simulink model "twiddle"  (R2018a)
settings: Solver=VariableStepAuto  StartTime=0.0  StopTime=10.0  RelTol=1e-3
undefined symbols (not defined in the file or in its folder): i
settings Model: Creator=berke  LastModifiedBy=berke

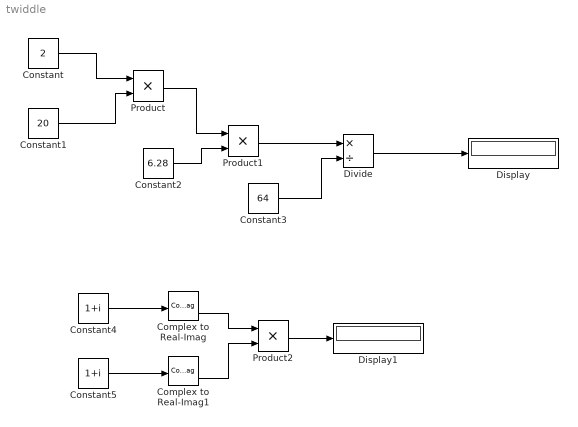
== system twiddle ==
  Complex to Real-Imag : ComplexToRealImag
  Complex to Real-Imag1 : ComplexToRealImag
  Constant : Constant  Value=2  OutDataTypeStr=fixdt(0,16,8)  SampleTime=0.1
  Constant1 : Constant  Value=20  OutDataTypeStr=fixdt(0,16,8)  SampleTime=0.1
  Constant2 : Constant  Value=6.28  OutMin=6.28  OutMax=6.28  OutDataTypeStr=fixdt(0,8,4)  SampleTime=0.1
  Constant3 : Constant  Value=64  OutDataTypeStr=fixdt(0,8,0)  SampleTime=0.1
  Constant4 : Constant  Value=1+i  SampleTime=0.1
  Constant5 : Constant  Value=1+i  SampleTime=0.1
  Display : Display
  Display1 : Display
  Divide : Product  Inputs=*/  SaturateOnIntegerOverflow=on  RndMeth=Zero
  Product : Product
  Product1 : Product
  Product2 : Product
  wires:
  Constant/1 -> Product/1
  Constant1/1 -> Product/2
  Product/1 -> Product1/1
  Constant2/1 -> Product1/2
  Product1/1 -> Divide/1
  Constant3/1 -> Divide/2
  Divide/1 -> Display/1
  Product2/1 -> Display1/1
  Constant4/1 -> Complex to Real-Imag/1
  Constant5/1 -> Complex to Real-Imag1/1
  Complex to Real-Imag1/2 -> Product2/2
  Complex to Real-Imag/2 -> Product2/1
